simulink model "Backups"  (R2020b)
settings: Solver=VariableStepAuto  StartTime=0.0  StopTime=10.0  RelTol=1e-3
undefined symbols (not defined in the file): O, P_Blowdown, P_Needleboi
libraries: pid_lib x3, simulink x1, dspfdesign x1
(part 2 of 2)

== matlab function Backups/MATLAB Function8 ==
  data: T input; dT output; dn_liq output; dn_vap output; m_dot output; nLiq input; nVap input; V input; m_tank input; Cd input; Pe input; A_inj input; P output; nPres input
function [dT, dn_liq, dn_vap, m_dot, P] = nox_blowdown(T, nLiq, nVap, V, m_tank, Cd, Pe, A_inj, nPres )
%OX_TANK_SIM Models thermochemical processes of blow-down in oxidizer tank.
%   Propellant Tank Pressurization Modeling for a Hybrid Rocket - Margaret
%   Mary Fernandez
%
%   INPUTS:
%       "n" = 1x2 vector of ox moles in tank (kmol).
%       "T" = ox tank temperature (K).
%       "V" = volume of ox tank (m^3).
%       "m_tank" = mass of oxidizer tank (kg).
%       "m_dot_prev" = ox mass flow rate of previous time step (kg/s).
%       "A_inj" = total orifice area of injector plate (m^2).
%       "Cd" = injector plate discharge coefficient.
%       "Pe" = pressure at exit of injector plate (Pa).
%
%   OUTPUTS:
%       "m_dot" = scalar ox mass flow rate (kg/s).
%       "dn" = 1x2 differential change in ox moles (kmol).
%       "dT" = differential change in ox tank temperature (K).
%       "P" = scalar internal pressure of ox tank (Pa).
%%%%%%%%%%%%%%%%%%%%%%%%%%%%%%%%%%%%%%%%%%%%%%%%%%%%%%%%%%%%%%%%%%%%%%%%%%%

%Perry's Chemical Engineers' Handbook Property Equations:
G1 = 96.512;           %Vapour pressure of N2O [Pa] coefficients
G2 = -4045;            % valid for Temp range [182.3 K - 309.57 K]
G3 = -12.277;
G4 = 2.886e-5;
G5 = 2;

Tc = 309.57;           % critical temperature of N2O [K]

J1 = 2.3215e7;         % heat of vaporization of N2O [J/kmol] coefficients
J2 = 0.384;            % valid for Temp range [182.3 K - 309.57 K]
J3 = 0;
J4 = 0;

% % heat capacity of N2 at constant pressure [J/(kmol*K)] coefficients
% % valid for Temp range [100 K - 1500 K]
% C1 = 0.28883e5; 
% C2 = 0;              
% C3 = 0;
% C4 = 0;
% C5 = 0;

D1 = 0.2934e5; % heat capacity of N2O gas at constant pressure [J/(kmol*K)] coefficients
D2 = 0.3236e5; % valid for Temp range [100 K - 1500 K]
D3 = 1.1238e3;
D4 = 0.2177e5;
D5 = 479.4; 

E1 = 6.7556e4; % heat capacity of N2O liquid at constant pressure [J/(kmol*K)] coefficients
E2 = 5.4373e1; % valid for Temp range [182.3 K - 200 K]
E3 = 0;
E4 = 0;
E5 = 0;
Q1 = 2.781;    % molar specific volume of liquid N2O [m^3/kmol] coefficients
Q2 = 0.27244;
Q3 = 309.57;
Q4 = 0.2882;

R  = 8314;      %Universal gas constant (J/kmol*K).
MW = 44.013;   %Molar mass of N2O (kg/kmol)​
% Calculate thermodynamic parameters as functions of temperature:
Vhat_l      = Q2^(1 + (1 - T/Q3)^Q4)/Q1;                    %Molar specific vol. of liq. N2O [m^3/kmol]
CVhat_g     = D1 + D2*((D3/T)/sinh(D3/T))^2 + ...
              D4*((D5/T)/cosh(D5/T))^2 - R;                 %Molar c_V of N2O gas [J/(kmol*K)]
CVhat_l     = E1 + E2*T + E3*T^2 + E4*T^3 + E5*T^4;         %Molar c_V of N2O liq.; approx. = c_P [J/(kmol*K)]
Tr          = T/Tc;                                         %Reduced temperature.
delta_Hv    = J1*(1 - Tr) ^ (J2 + J3*Tr + J4*Tr^2);         %Heat of vaporization of N2O [J/kmol]
P_sat       = exp(G1 + G2/T + G3*log(T) + G4*T^G5);         %Vapour P of N20 (Pa).
dP_sat      = (-G2/(T^2) + G3/T + G4*G5*T^(G5-1)) ...       %Derivative of vapour P with respect to T.
              * exp(G1 + G2/T + G3*log(T) + G4*T^G5);        
c_P         = (4.8 + 0.00322*T)*155.239;                    %Specific heat of tank, Aluminum [J/kg*K]


%Simplified expression definitions for solution:
P = (nPres+nVap)*R*T/(V - nLiq*Vhat_l);
a = m_tank*c_P  + nPres*CVhat_l+nVap*CVhat_g + nLiq*CVhat_l;
RT = P*Vhat_l;
e = -delta_Hv + R*T;
f = -Cd*A_inj*sqrt(abs(2/MW*(P - Pe)/Vhat_l));
j = -Vhat_l*P_sat;
k = (V - nLiq*Vhat_l)*dP_sat;
l = R*T;
q = R*nVap;
Z = (-f*(-j*a + (q - k)*RT))/(a*(l + j) + (q - k)*(e - RT));
W = (-Z*(l*a + (q - k)*e))/(-j*a + (q - k)*RT);
%Time derivative of tank conditions
m_dot = -f*MW;          % Mass flow rate
dn_liq    = W;    % Time derivative of nitrous amount
dn_vap=Z;
dT    = (RT*W + e*Z)/a;  % Time derivative of tank temperature

end

== matlab function Backups/Needle Valve1/Area of Orfice/Orfice Area ==
  data: A_leak input; A_Orf output; Orf_diam input; theta input; h input; h_max output
function [A_Orf, h_max] = OrficeArea(A_leak, Orf_diam, theta, h)
h_max=(Orf_diam*(1-sqrt(1-cos(theta/2))))/sin(theta);

if (h<=0)
    A_Orf= A_leak;
elseif (h>0) && (h<h_max)
    A_Orf=(pi*(Orf_diam-(h*sin(theta/2)*cos(theta/2)))*h*sin(theta/2))+A_leak;
elseif (h>h_max)
    A_Orf=(pi*(Orf_diam)^2/4)+A_leak;
else
    A_Orf=(pi*(Orf_diam)^2/4)+A_leak;
end

%A_Orf=(pi*(Orf_diam)^2/4)+A_leak;

== matlab function Backups/Subsystem/MATLAB Function ==
  data: P input; T input; dZdT output; dZdP output; Z output
function [dZdT, dZdP, Z]  = get_dZ_N2(P, T)

    P           = P / 6894.76;
    
    nh_theta    = [0.90370032155133;...
                          -3.99164830787538;...
                           4.44554878990612;...
                          -1.68387394930366;...
                           1.84282855081908;...
                          -2.71807522455834;...
                           1.80658523674363;...
                          -0.00026662830718;...
                           0.16405364316350];

    nh_alpha    = [1;               ...
                           0.45607085009281;...
                           0.99224794564113;...
                           1.58495789262624;...
                           0.53133147588636;...
                           1.29132167947510;...
                           1.44008913900161;...
                           2.74997487910292;...
                           2.36611999082672];

    nl_theta    = [0.46742656471647;...
                          -0.53799565472298;...
                          -9.22454428760102;...
                           9.15603503101003;...
                           3.18808664459882;...
                           0.30163700042055;...
                          -0.27300234680706;...
                          -1.00749719408221;...
                          -1.49106816983329];

    nl_alpha    = [1;               ...
                           1.41102397459172;...
                           0.33562799290636;...
                           0.79810083070486;...
                           0.01008992455881;...
                           2.53968667359886;...
                           2.51281397715323;...
                           1.20879498088509;...
                           1.69572064361084];
                       
    if (T >= 220 && T <= 320) && (P >= 800 && P <= 4500)

        T           = T / 126.2;
        P           = P / 492.3;

        dZdTr       = nh_theta(2)*nh_alpha(2)*T^(nh_alpha(2) - 1)*P^0.7   ...
                    + nh_theta(3)*nh_alpha(3)*T^(nh_alpha(3) - 1)*P^0.5   ...
                    + nh_theta(4)*nh_alpha(4)*T^(nh_alpha(4) - 1)*P^0.3   ...
                    + nh_theta(5)*nh_alpha(5)*T^(nh_alpha(5) - 1)*P       ...
                    + nh_theta(6)*nh_alpha(6)*T^(nh_alpha(6) - 1)*P       ...
                    + nh_theta(7)*nh_alpha(7)*T^(nh_alpha(7) - 1)*P       ...
                    + nh_theta(9)*nh_alpha(9)*T^(nh_alpha(9) - 1);

        dZdT        = dZdTr / 126.2;

        dZdPr       = 0.7*nh_theta(2)*T^nh_alpha(2)*P^(-0.3)        ...
                    + 0.5*nh_theta(3)*T^nh_alpha(3)*P^(-0.5)        ...
                    + 0.3*nh_theta(4)*T^nh_alpha(4)*P^(-0.7)        ...
                    + nh_theta(5)*T^nh_alpha(5)                     ...
                    + nh_theta(6)*T^nh_alpha(6)                     ...
                    + nh_theta(7)*T^nh_alpha(7)                     ...
                    + nh_theta(8)*nh_alpha(8)*P^(nh_alpha(8) - 1);

        dZdP        = dZdPr / 492.3;     

        N           = [1;                       ...
                        T^nh_alpha(2)*P^0.7;     ...
                        T^nh_alpha(3)*P^0.5;     ...
                        T^nh_alpha(4)*P^0.3;     ...
                        T^nh_alpha(5)*P;           ...
                        T^nh_alpha(6)*P;           ...
                        T^nh_alpha(7)*P;           ...
                        P^nh_alpha(8);             ...
                        T^nh_alpha(9)];               

        Z       = sum(nh_theta .* N);        

    elseif (T >= 180 && T < 220) && (P >= 800 && P <= 4500)

        T           = T / 126.2;
        P           = P / 492.3;

        dZdTr       = nl_theta(2)*nl_alpha(2)*T^(nl_alpha(2) - 1)*P^0.7   ...
                    + nl_theta(3)*nl_alpha(3)*T^(nl_alpha(3) - 1)*P^0.5   ...
                    + nl_theta(4)*nl_alpha(4)*T^(nl_alpha(4) - 1)*P^0.3   ...
                    + nl_theta(5)*nl_alpha(5)*T^(nl_alpha(5) - 1)*P       ...
                    + nl_theta(6)*nl_alpha(6)*T^(nl_alpha(6) - 1)*P       ...
                    + nl_theta(7)*nl_alpha(7)*T^(nl_alpha(7) - 1)*P       ...
                    + nl_theta(9)*nl_alpha(9)*T^(nl_alpha(9) - 1);

        dZdT        = dZdTr / 126.2;

        dZdPr       = 0.7*nl_theta(2)*T^nl_alpha(2)*P^(-0.3)        ...
                    + 0.5*nl_theta(3)*T^nl_alpha(3)*P^(-0.5)        ...
                    + 0.3*nl_theta(4)*T^nl_alpha(4)*P^(-0.7)        ...
                    + nl_theta(5)*T^nl_alpha(5)                     ...
                    + nl_theta(6)*T^nl_alpha(6)                     ...
                    + nl_theta(7)*T^nl_alpha(7)                     ...
                    + nl_theta(8)*nl_alpha(8)*P^(nl_alpha(8) - 1);

        dZdP        = dZdPr / 492.3;     

        N           = [1;                       ...
                        T^nl_alpha(2)*P^0.7;     ...
                        T^nl_alpha(3)*P^0.5;     ...
                        T^nl_alpha(4)*P^0.3;     ...
                        T^nl_alpha(5)*P;           ...
                        T^nl_alpha(6)*P;           ...
                        T^nl_alpha(7)*P;           ...
                        P^nl_alpha(8);             ...
                        T^nl_alpha(9)];               

        Z       = sum(nl_theta .* N); 

    else
        T           = 180 / 126.2;
        P           = P / 492.3;

        dZdTr       = nl_theta(2)*nl_alpha(2)*T^(nl_alpha(2) - 1)*P^0.7   ...
                    + nl_theta(3)*nl_alpha(3)*T^(nl_alpha(3) - 1)*P^0.5   ...
                    + nl_theta(4)*nl_alpha(4)*T^(nl_alpha(4) - 1)*P^0.3   ...
                    + nl_theta(5)*nl_alpha(5)*T^(nl_alpha(5) - 1)*P       ...
                    + nl_theta(6)*nl_alpha(6)*T^(nl_alpha(6) - 1)*P       ...
                    + nl_theta(7)*nl_alpha(7)*T^(nl_alpha(7) - 1)*P       ...
                    + nl_theta(9)*nl_alpha(9)*T^(nl_alpha(9) - 1);

        dZdT        = dZdTr / 126.2;

        dZdPr       = 0.7*nl_theta(2)*T^nl_alpha(2)*P^(-0.3)        ...
                    + 0.5*nl_theta(3)*T^nl_alpha(3)*P^(-0.5)        ...
                    + 0.3*nl_theta(4)*T^nl_alpha(4)*P^(-0.7)        ...
                    + nl_theta(5)*T^nl_alpha(5)                     ...
                    + nl_theta(6)*T^nl_alpha(6)                     ...
                    + nl_theta(7)*T^nl_alpha(7)                     ...
                    + nl_theta(8)*nl_alpha(8)*P^(nl_alpha(8) - 1);

        dZdP        = dZdPr / 492.3;  

    N           = [1;                       ...
                    T^nl_alpha(2)*P^0.7;     ...
                    T^nl_alpha(3)*P^0.5;     ...
                    T^nl_alpha(4)*P^0.3;     ...
                    T^nl_alpha(5)*P;           ...
                    T^nl_alpha(6)*P;           ...
                    T^nl_alpha(7)*P;           ...
                    P^nl_alpha(8);             ...
                    T^nl_alpha(9)];               

    Z       = sum(nl_theta .* N); 

    end
end

== matlab function Backups/n2_blow ==
  data: mdot input; T input; P input; Z input; Zt input; Zb input; m input; V input; dPdt output; qdot input; dTdt output
function [dPdt, dTdt] = n2_blowdown(mdot, T, P, Z, Zt, Zb, m, V, qdot)

    R = 8314 / 28;
    cnv = 6894.76;

    Zp = Zb/cnv;
    cv = 776;

    dPdt = (m*R*Z^2 + P*V*Zt)*qdot/(V*cv*(m*(Z - P*Zp)))    ...
         - mdot*((cv + Z*R)*m*Z + P*V*Zt)*(P/(m*cv))/(m*(Z - P*Zp));

    dZdt = (m*R*Z^2 * Zp + V*Z*Zt)*dPdt/(m*R*Z^2 + P*V)     ...
         - Zt*(P*V*Z/m)*mdot/(m*R*Z^2 + P*V);

    dTdt = V*(dPdt/(m*Z) - dZdt*P/(m*Z^2) - mdot*P/(m*Z^2))/R;
end

== matlab function Backups/MATLAB Function ==
  data: A_inj output; m_dot_des input
function A_inj  = A_inj(m_dot_des)
Cd=0.650000000000000;
MW=350000;
P=100;
Pe=50;
Vhat_l=0.12;

A_inj=(m_dot_des)/(Cd*sqrt(abs(2/MW*(P - Pe)/Vhat_l))*MW);

== matlab function Backups/MATLAB Function2 ==
  data: dn output; n input; m_dot output; T input; V input; m_tank input; A_inj input; Cd input; Pe input; nPres input; dT output; P output
function [dn,m_dot, dT, P] = CoolPropTest(n, T, V, m_tank, A_inj, Cd, Pe, nPres)
P=100000;
%OX_TANK_SIM Models thermochemical processes of blow-down in oxidizer tank.
%   Propellant Tank Pressurization Modeling for a Hybrid Rocket - Margaret
%   Mary Fernandez
%
%   INPUTS:
%       "n" = 1x2 vector of ox moles in tank (kmol).
%       "T" = ox tank temperature (K).
%       "V" = volume of ox tank (m^3).
%       "m_tank" = mass of oxidizer tank (kg).
  %    "m_dot_prev" = ox mass flow rate of previous time step (kg/s).
%       "A_inj" = total orifice area of injector plate (m^2).
%       "Cd" = injector plate discharge coefficient.
%       "Pe" = pressure at exit of injector plate (Pa).
%
%   OUTPUTS:
%       "m_dot" = scalar ox mass flow rate (kg/s).
%       "dn" = 1x2 differential change in ox moles (kmol).
%       "dT" = differential change in ox tank temperature (K).
%       "P" = scalar internal pressure of ox tank (Pa).
%%%%%%%%%%%%%%%%%%%%%%%%%%%%%%%%%%%%%%%%%%%%%%%%%%%%%%%%%%%%%%%%%%%%%%%%%%%


R  = 8314;
MW = 44.013;   %Molar mass of N2O (kg/kmol).
T=298;
            

                % Molar specific vol. of liq. N2O [m^3/kmol]
                Vhat_l      = MW / py.CoolProp.CoolProp.PropsSI('D', 'P', P(1), 'T', T(1), 'N2O');

                % Molar c_V of Pressurant gas [J/(kmol*K)]
                CVhat_Pres  =MW * py.CoolProp.CoolProp.PropsSI('O', 'P', P(1), 'T', T(1));

                % Molar c_V of N2O gas [J/(kmol*K)]
                CVhat_g     = MW * py.CoolProp.CoolProp.PropsSI('O', 'T', T(1), 'Q', 1, 'N2O') - R;

                % Molar c_V of N2O liq approx. = c_P [J/(kmol*K)]
                CVhat_l     = MW * py.CoolProp.CoolProp.PropsSI('C', 'T', T(1), 'Q', 1, 'N2O');

                % Heat of vaporization of N2O [J/kmol]
                Hv          = py.CoolProp.CoolProp.PropsSI('H', 'T', T(1), 'Q', 1, 'N2O');
                Hl          = py.CoolProp.CoolProp.PropsSI('H', 'T', T(1), 'Q', 0, 'N2O');
                delta_Hv    = MW * (Hv - Hl);

                % Vapour P of N20 (Pa).
                P_sat       = py.CoolProp.CoolProp.PropsSI('P', 'T', T(1), 'Q', 0, 'N2O');

                % Derivative of vapour P with respect to T.
                dP_sat      = py.CoolProp.CoolProp.PropsSI('d(P)/d(T)|D', 'T', T, 'Q', 1, 'N2O');
               
                c_P         = (4.8 + 0.00322*T)*155.239;                    %Specific heat of tank, Aluminum [J/kg*K]


            P           = (nPres + n(2))*obj.utilities.R*T/(V - n(1)*Vhat_l);
            a           = m_tank*c_P + nPres*CVhat_Pres + n(2)*CVhat_g + n(1)*CVhat_l;
            RT          = P*Vhat_l;
            e           = -delta_Hv + RT;
            f           = -Cd*A_inj*sqrt(abs(2/MW*(P - Pe)/Vhat_l));
            j           = -Vhat_l*P_sat;
            k           = (V- n(1)*Vhat_l)*dP_sat;
            l           = R*T;
            q           = R*n(2);

            Z           = (-f*(-j*a + (q - k)*RT))/(a*(l + j) + (q - k)*(e - RT));
            W           = (-Z*(l*a + (q - k)*e))/(-j*a + (q - k)*RT);

            dT          = (RT*W + e*Z)/a;
            


%Time derivative of tank conditions
            m_dot     = -f*MW;         % Mass flow rate
            dn       = [W, Z];                       % Time derivative of nitrous amount
            dT       = [dT, dT];                     % Time derivative of tank temperature

end

== matlab function Backups/Needle Valve1/Valve Region/Valve Region ==
  data: rho input; q output; p1 input; del_P output; p2 input; Re_crit input; visc input; A_Orf input; Cd input
function[q, del_P] = NeedleValve(rho,p1,p2, Re_crit, visc,A_Orf,Cd)
% theta= angle of tip of needle assuming 90 initially later can be created
% as workspace variable
%h_init = initial height of needle (not 0 prolly for all practical purposes)
%Orf_diam is the diameter of the orfice
%Re_crit is the critical reynolds number
%q is the mass flow rate
%visc = fluid kinematic viscosity
%del_P is the pressure differential

del_P=p1-p2;
Dh=sqrt((4*A_Orf)/pi);
P_minT=(rho/2)*((Re_crit*visc)/(Cd*Dh))^2;
q=Cd*A_Orf*sqrt(2/rho)*del_P/((((del_P))^2+(P_minT)^2))^0.25;
%del_P=6894.76*5.4*10^(-7)*rho*;

== matlab function Backups/Cv1 ==
  data: Cv output; u input
function Cv = Cvcalc(u)
if (u<6)
    Cv = u/20;
elseif(u>6&&u<9)
Cv=((1.1169*(u-5.95)^2))/10+0.3;
else
  Cv=0;
    
end

== matlab function Backups/Input_Blowdown/A_injector/MATLAB Function1 ==
  data: A_inj output; m_dot_des input
function A_inj  = A_inj(m_dot_des)
Cd=0.50;
MW=44;
P=3.62e6;
Pe=2.413e6;
Vhat_l=0.05;

A_inj=(m_dot_des)/(Cd*sqrt(abs(2/MW*(P - Pe)/Vhat_l))*MW);

== matlab function Backups/Needle Valve3/Orfice Area ==
  data: A_leak input; A_Orf output; Orf_diam input; theta input; h input; h_max output
function [A_Orf, h_max] = OrficeArea(A_leak, Orf_diam, theta, h)
h_max=(Orf_diam*(1-sqrt(1-cos(theta/2))))/sin(theta);

if (h<=0)
    A_Orf= A_leak;
elseif (h>0) && (h<h_max)
    A_Orf=(pi*(Orf_diam-(h*sin(theta/2)*cos(theta/2)))*h*sin(theta/2))+A_leak;
elseif (h>h_max)
    A_Orf=(pi*(Orf_diam)^2/4)+A_leak;
else
    A_Orf=(pi*(Orf_diam)^2/4)+A_leak;
end

%A_Orf=(pi*(Orf_diam)^2/4)+A_leak;

== matlab function Backups/Needle Valve3/Valve Region1 ==
  data: rho input; q output; p1 input; del_P output; p2 input; Re_crit input; visc input; A_Orf input; Cd input
function[q, del_P] = NeedleValve(rho,p1,p2, Re_crit, visc,A_Orf,Cd)
% theta= angle of tip of needle assuming 90 initially later can be created
% as workspace variable
%h_init = initial height of needle (not 0 prolly for all practical purposes)
%Orf_diam is the diameter of the orfice
%Re_crit is the critical reynolds number
%q is the mass flow rate
%visc = fluid kinematic viscosity
%del_P is the pressure differential

Dh=sqrt((4*A_Orf)/pi);
del_P=p1-p2;
P_minT=(rho/2)*((Re_crit*visc)/(Cd*Dh))^2;
q=Cd*A_Orf*sqrt(2/rho)*del_P/((((del_P))^2+(P_minT)^2))^0.25;
